simulink model "rig_real_time_template_2023"  (R2023b)
settings: Solver=ode1  StartTime=0.0  StopTime=60  RelTol=1e-3  EnableMultiTasking=on
values from neighbouring files (symbols this model uses):
  den1 = cell2mat(HY3_N1_D.denominator)    [ThreeDiskOscillator.m]
  den2 = cell2mat(HY3_N2_D.denominator)    [ThreeDiskOscillator.m]
  num_HY1_N1_D = cell2mat(HY1_N1_D.numerator)    [ThreeDiskOscillator.m]
  num_HY2_N1_D = cell2mat(HY2_N1_D.numerator)    [ThreeDiskOscillator.m]
  num_HY2_N2_D = cell2mat(HY2_N2_D.numerator)    [ThreeDiskOscillator.m]
  num_HY3_N1_D = cell2mat(HY3_N1_D.numerator)    [ThreeDiskOscillator.m]
  num_HY3_N2_D = cell2mat(HY3_N2_D.numerator)    [ThreeDiskOscillator.m]
undefined symbols (not defined in the file or in its folder): M
settings Model: SimulationMode=external  ExtModeTrigDuration=75001  Creator=Dro  LastModifiedBy=andre
settings SolverCC: AlgebraicLoopSolver=TrustRegion
settings DataIOCC: LimitDataPoints=on  SaveFormat=Array  ReturnWorkspaceOutputs=off  SignalLoggingName=sigsOut
settings OptimizationCC: ExpressionDepthLimit=2147483647  InitFltsAndDblsToZero=on
settings DebuggingCC: SaveWithParameterizedLinksMsg=none  UnderspecifiedInitializationDetection=Classic  MergeDetectMultiDrivingBlocksExec=none  SignalResolutionControl=TryResolveAllWithWarning  MultiTaskDSMMsg=warning  MultiTaskCondExecSysMsg=none  FcnCallInpInsideContextMsg=warning  UnconnectedInputMsg=warning  UnconnectedOutputMsg=warning  UnconnectedLineMsg=warning  StateNameClashWarn=warning  SFUnexpectedBacktrackingDiag=warning  SFNoUnconditionalDefaultTransitionDiag=warning  SFExecutionAtInitializationDiag=none  ArithmeticOperatorsInVariantConditions=warning
settings HardwareCC: ProdBitPerLong=64  ProdHWDeviceType=Intel->x86-64 (Linux 64)
settings ModelReferenceCC: EnableRefExpFcnMdlSchedulingChecks=on  PropagateSignalLabelsOutOfModel=off
settings SFSimCC: SimUseLocalCustomCode=off  CustomCodeUndefinedFunction=UseInterfaceOnly
settings RTWCC: Description=Simulink Desktop Real-Time  SystemTargetFile=sldrt.tlc  TemplateMakefile=sldrt.tmf  RTWUseLocalCustomCode=off  RTWCompilerOptimization=on
settings CodeAppCC: MaxIdLength=95  StateflowObjectComments=on
settings SimulinkDesktopRealTimeCC: TargetLibSuffix=_sldrt.a  TargetPreCompLibLocation=C:\Program Files\MATLAB\R2023b\toolbox\sldrt\lib\win64  TargetLangStandard=C89/C90 (ANSI)
settings ConfigComp: CovMetricSettings=dw  CovSaveCumulativeToWorkspaceVar=on  CovSaveSingleToWorkspaceVar=on  CovExternalEMLEnable=off

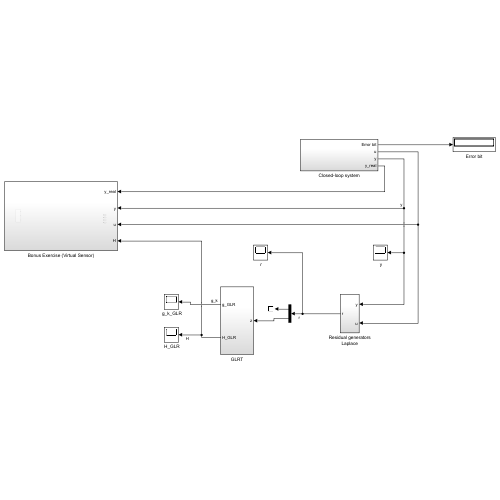
[thumbnail: Simulink's stored preview of the top-level diagram]
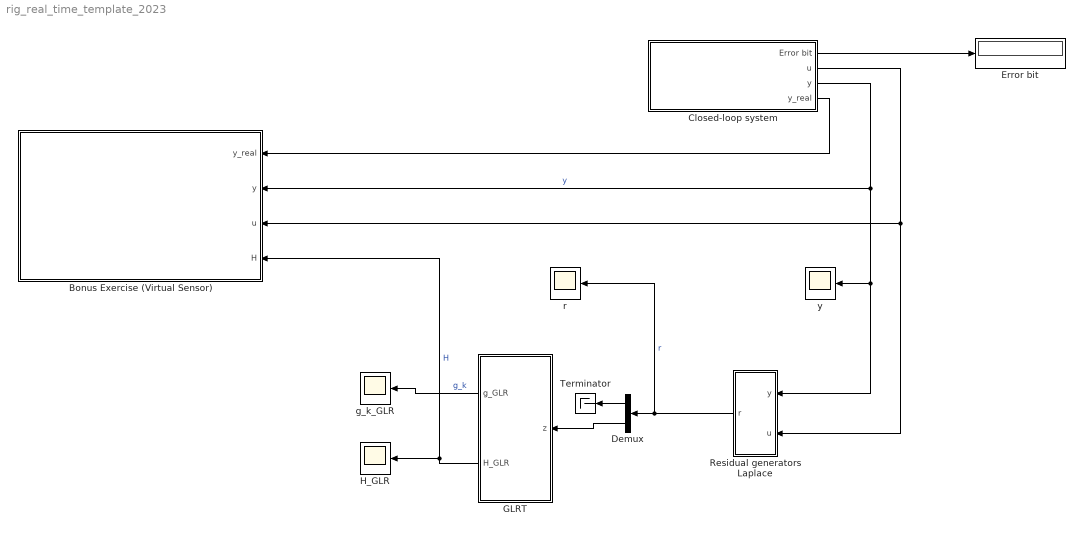
== system rig_real_time_template_2023 ==
  " H_GLR" : Scope
  " g_k_GLR" : Scope
  " r" : Scope
  " y" : Scope
  Bonus Exercise (Virtual Sensor) : Subsystem
  Closed-loop system : Subsystem
  Demux : Demux  Outputs=2
  "Error bit " : Display
  GLRT : Subsystem
  Residual generators Laplace : Subsystem
  Terminator : Terminator
  wires:
  Closed-loop system/2(u) -> Residual generators Laplace/2(u), Bonus Exercise (Virtual Sensor)/3(u)
  Closed-loop system/1(Error bit) -> "Error bit "/1
  Residual generators Laplace/1(r) -> Demux/1, " r"/1  "r"
  Closed-loop system/3(y) -> Residual generators Laplace/1(y), " y"/1, Bonus Exercise (Virtual Sensor)/2(y)  "y"
  GLRT/1(g_GLR) -> " g_k_GLR"/1  "g_k"
  GLRT/2(H_GLR) -> Bonus Exercise (Virtual Sensor)/4(H), " H_GLR"/1  "H"
  Closed-loop system/4(y_real) -> Bonus Exercise (Virtual Sensor)/1(y_real)
  Demux/2 -> GLRT/1(z)
  Demux/1 -> Terminator/1

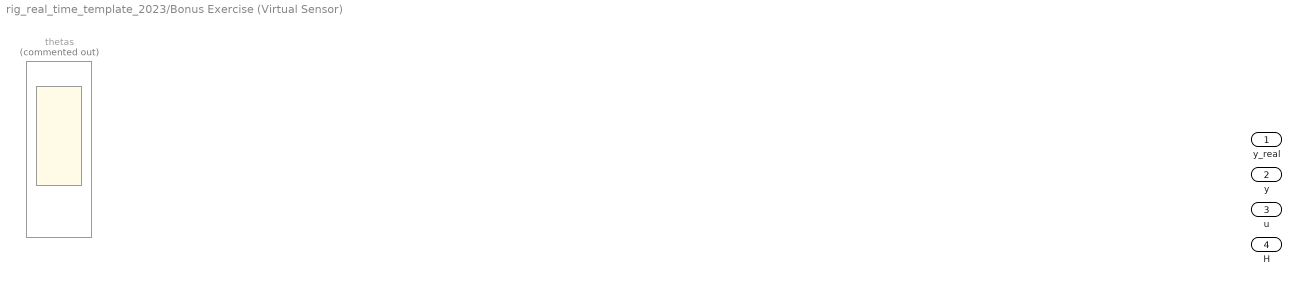
== system rig_real_time_template_2023/Bonus Exercise (Virtual Sensor) ==
  y_real : Inport
  y : Inport  Port=2
  u : Inport  Port=3
  H : Inport  Port=4
  thetas : Scope  Commented=on  NumInputPorts=3

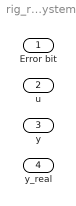
== system rig_real_time_template_2023/Closed-loop system ==
  Error bit : Outport  VectorParamsAs1DForOutWhenUnconnected=off
  u : Outport  Port=2  VectorParamsAs1DForOutWhenUnconnected=off
  y : Outport  Port=3  VectorParamsAs1DForOutWhenUnconnected=off
  y_real : Outport  Port=4  VectorParamsAs1DForOutWhenUnconnected=off

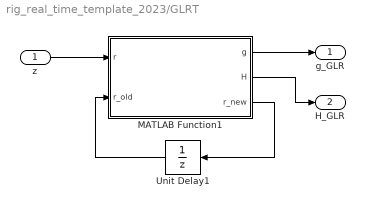
== system rig_real_time_template_2023/GLRT ==
  z : Inport
  MATLAB Function1 : MATLAB Function  TreatAsAtomicUnit=on
  Unit Delay1 : UnitDelay  InitialCondition=zeros(M-1,1)  SampleTime=-1  HasFrameUpgradeWarning=on
  g_GLR : Outport  VectorParamsAs1DForOutWhenUnconnected=off
  H_GLR : Outport  Port=2  VectorParamsAs1DForOutWhenUnconnected=off
  wires:
  MATLAB Function1/3(r_new) -> Unit Delay1/1
  Unit Delay1/1 -> MATLAB Function1/2(r_old)
  z/1 -> MATLAB Function1/1(r)
  MATLAB Function1/1(g) -> g_GLR/1
  MATLAB Function1/2(H) -> H_GLR/1

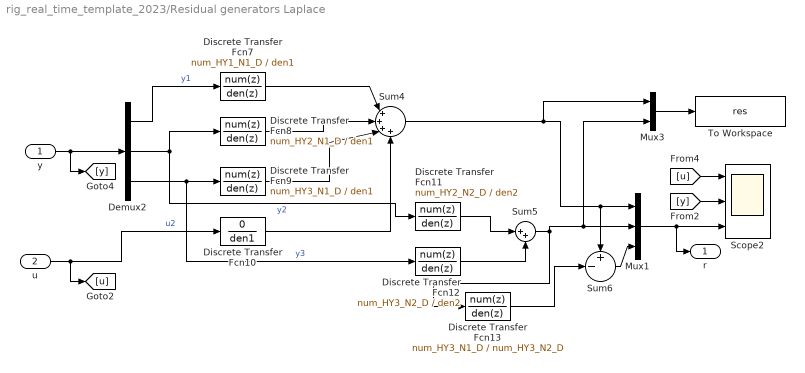
== system rig_real_time_template_2023/Residual generators Laplace ==
  y : Inport
  u : Inport  Port=2
  Demux2 : Demux  Outputs=3
  Discrete Transfer Fcn10 : DiscreteTransferFcn  Numerator=0  Denominator=den1
  Discrete Transfer Fcn11 : DiscreteTransferFcn  Numerator=num_HY2_N2_D  Denominator=den2
  Discrete Transfer Fcn12 : DiscreteTransferFcn  Numerator=num_HY3_N2_D  Denominator=den2
  Discrete Transfer Fcn13 : DiscreteTransferFcn  Numerator=num_HY3_N1_D  Denominator=num_HY3_N2_D
  Discrete Transfer Fcn7 : DiscreteTransferFcn  Numerator=num_HY1_N1_D  Denominator=den1
  Discrete Transfer Fcn8 : DiscreteTransferFcn  Numerator=num_HY2_N1_D  Denominator=den1
  Discrete Transfer Fcn9 : DiscreteTransferFcn  Numerator=num_HY3_N1_D  Denominator=den1
  Mux1 : Mux  Inputs=3
  Mux3 : Mux  Inputs=2
  Scope2 : Scope  NumInputPorts=3
  Sum4 : Sum  Inputs=|++++
  Sum5 : Sum  Inputs=|++
  Sum6 : Sum  Inputs=+-|
  To Workspace : ToWorkspace  VariableName=res  SaveFormat=Structure With Time  SampleTime=-1
  r : Outport  VectorParamsAs1DForOutWhenUnconnected=off
  wires:
  Sum4/1 -> Mux3/1, Mux1/1, Sum6/1
  Mux1/1 -> r/1, Scope2/3
  y/1 -> [y], Demux2/1
  Sum5/1 -> Mux3/2, Mux1/2, Discrete Transfer Fcn13/1
  Demux2/1 -> Discrete Transfer Fcn7/1  "y1"
  Discrete Transfer Fcn11/1 -> Sum5/1
  Discrete Transfer Fcn13/1 -> Sum6/2
  Sum6/1 -> Mux1/3
  Discrete Transfer Fcn10/1 -> Sum4/4
  Demux2/2 -> Discrete Transfer Fcn8/1, Discrete Transfer Fcn11/1  "y2"
  Discrete Transfer Fcn12/1 -> Sum5/2
  u/1 -> Discrete Transfer Fcn10/1, [u]  "u2"
  [u] -> Scope2/1
  [y] -> Scope2/2
  Discrete Transfer Fcn9/1 -> Sum4/3
  Mux3/1 -> To Workspace/1
  Demux2/3 -> Discrete Transfer Fcn12/1, Discrete Transfer Fcn9/1  "y3"
  Discrete Transfer Fcn7/1 -> Sum4/1
  Discrete Transfer Fcn8/1 -> Sum4/2

== matlab function rig_real_time_template_2023/GLRT/MATLAB Function1 ==
  data: r input; g output size=1; H output; r_old input; r_new output
function [g, H, r_new] = GLR(r, r_old)

h = 7.568;          % h from workspace
sigma = 0.0010662;  % Sigma from workspace
M  = 10;            % M from workspace

z = [r_old(2:end); r];    % Concatenate data

maxsum = 0;
sumin=(sum(z))^2;
for j = 1:M
    sumin=(sum(z))^2;
    if sumin > maxsum
        maxsum = sumin;
    end
end
g = 1/(2 * sigma * M) * maxsum;

if g >= h
    H = 1;
else
    H = 0;
end

r_new = z(9,:);

end
